simulink model "unicycle"  (R2025b)
settings: Solver=VariableStepAuto  StartTime=0.0  StopTime=10.0  RelTol=1e-3
settings Model: Creator=nyanklc  LastModifiedBy=noyan

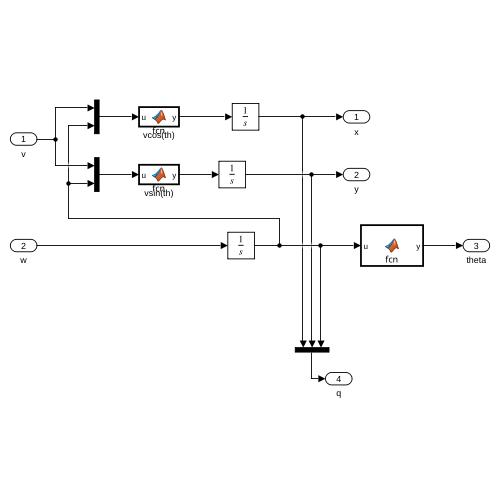
[thumbnail: Simulink's stored preview of the top-level diagram]
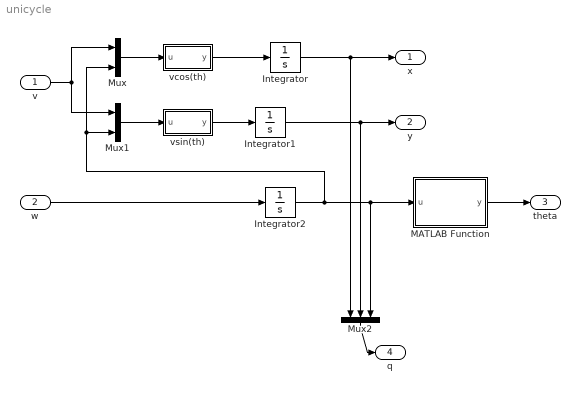
== system unicycle ==
  v : Inport
  w : Inport  Port=2
  Integrator : Integrator
  Integrator1 : Integrator
  Integrator2 : Integrator
  MATLAB Function : MATLAB Function  TreatAsAtomicUnit=on
  Mux : Mux  Inputs=2
  Mux1 : Mux  Inputs=2
  Mux2 : Mux  Inputs=3
  vcos(th) : MATLAB Function  TreatAsAtomicUnit=on
  vsin(th) : MATLAB Function  TreatAsAtomicUnit=on
  x : Outport
  y : Outport  Port=2
  theta : Outport  Port=3
  q : Outport  Port=4
  wires:
  Integrator/1 -> x/1, Mux2/1
  Integrator1/1 -> y/1, Mux2/2
  Integrator2/1 -> Mux/2, Mux1/2, MATLAB Function/1(u), Mux2/3
  w/1 -> Integrator2/1
  vcos(th)/1(y) -> Integrator/1
  Mux/1 -> vcos(th)/1(u)
  v/1 -> Mux1/1, Mux/1
  vsin(th)/1(y) -> Integrator1/1
  Mux1/1 -> vsin(th)/1(u)
  Mux2/1 -> q/1
  MATLAB Function/1(y) -> theta/1

== matlab function unicycle/vcos(th) ==
  data: u input; y output
function y = fcn(u)
v = u(1);
theta = u(2);
y = v * cos(theta);

== matlab function unicycle/MATLAB Function ==
  data: u input; y output
function y = fcn(u)

y = wrapToPi(u);

== matlab function unicycle/vsin(th) ==
  data: u input; y output
function y = fcn(u)
v = u(1);
theta = u(2);
y = v * sin(theta);
